simulink model "tvc"  (R2021a)
settings: Solver=VariableStepAuto  StartTime=0.0  StopTime=5  RelTol=1e-3
libraries: simulink_extras x1, simulink x1
settings Model: Creator=shohei  LastModifiedBy=shohei

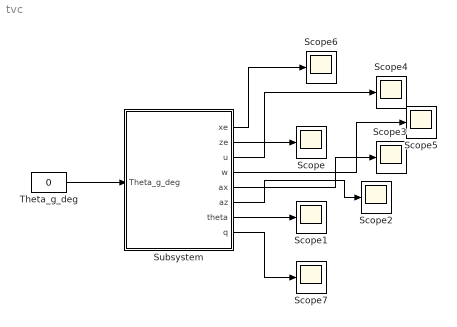
== system tvc ==
  Scope{,1..7} (8 alike) : Scope
  Subsystem : Subsystem
  Theta_g_deg : Constant  Value=0
  wires:
  Theta_g_deg/1 -> Subsystem/1(Theta_g_deg)
  Subsystem/2(ze) -> Scope/1
  Subsystem/7(theta) -> Scope1/1
  Subsystem/6(az) -> Scope2/1
  Subsystem/5(ax) -> Scope3/1
  Subsystem/3(u) -> Scope4/1
  Subsystem/4(w) -> Scope5/1
  Subsystem/1(xe) -> Scope6/1
  Subsystem/8(q) -> Scope7/1

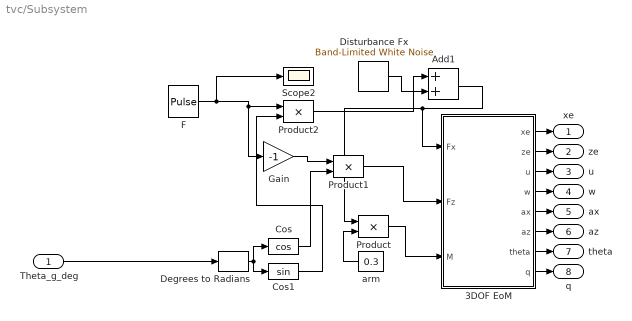
== system tvc/Subsystem ==
  Theta_g_deg : Inport
  3DOF EoM : Subsystem
  Add1 : Sum
  Cos : Trigonometry  Operator=cos
  Cos1 : Trigonometry
  Degrees to Radians : simulink_extras/Transformations/Degrees to Radians
  Disturbance Fx : simulink/Sources/Band-Limited White Noise  Cov=[0.001]  Ts=0.1  seed=[13342]
  F : DiscretePulseGenerator  PulseType=Time based  Amplitude=10  Period=100
  Gain : Gain  Gain=-1
  Product : Product
  Product1 : Product
  Product2 : Product
  Scope2 : Scope
  arm : Constant  Value=0.3
  xe : Outport
  ze : Outport  Port=2
  u : Outport  Port=3
  w : Outport  Port=4
  ax : Outport  Port=5
  az : Outport  Port=6
  theta : Outport  Port=7
  q : Outport  Port=8
  wires:
  3DOF EoM/8(q) -> q/1
  3DOF EoM/6(az) -> az/1
  3DOF EoM/7(theta) -> theta/1
  3DOF EoM/1(xe) -> xe/1
  3DOF EoM/3(u) -> u/1
  3DOF EoM/5(ax) -> ax/1
  Cos1/1 -> Product2/2
  3DOF EoM/4(w) -> w/1
  Product/1 -> 3DOF EoM/3(M)
  3DOF EoM/2(ze) -> ze/1
  Gain/1 -> Product1/1
  Theta_g_deg/1 -> Degrees to Radians/1
  arm/1 -> Product/2
  F/1 -> Gain/1, Product2/1, Scope2/1
  Degrees to Radians/1 -> Cos1/1, Cos/1
  Cos/1 -> Product1/2
  Add1/1 -> Product/1, 3DOF EoM/1(Fx)
  Product2/1 -> Add1/1
  Disturbance Fx/1 -> Add1/2
  Product1/1 -> 3DOF EoM/2(Fz)

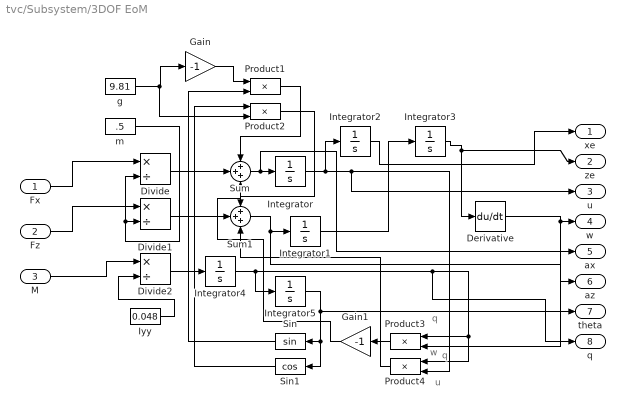
== system tvc/Subsystem/3DOF EoM ==
  note: w
  note: u
  note: q
  note: q
  Fx : Inport
  Fz : Inport  Port=2
  M : Inport  Port=3
  Derivative : Derivative
  Divide : Product  Inputs=*/
  Divide1 : Product  Inputs=*/
  Divide2 : Product  Inputs=*/
  Gain : Gain  Gain=-1
  Gain1 : Gain  Gain=-1
  Integrator{,1..2,4..5} (5 alike) : Integrator
  Integrator3 : Integrator  LimitOutput=on  UpperSaturationLimit=0
  Iyy : Constant  Value=0.048
  Product{1..4} (4 alike) : Product
  Sin : Trigonometry
  Sin1 : Trigonometry  Operator=cos
  Sum : Sum  Inputs=+++
  Sum1 : Sum  Inputs=+++
  g : Constant  Value=9.81
  m : Constant  Value=.5
  xe : Outport
  ze : Outport  Port=2
  u : Outport  Port=3
  w : Outport  Port=4
  ax : Outport  Port=5
  az : Outport  Port=6
  theta : Outport  Port=7
  q : Outport  Port=8
  wires:
  Fz/1 -> Divide1/1
  Gain/1 -> Product1/1
  Divide2/1 -> Integrator4/1
  m/1 -> Divide/2, Divide1/2
  Integrator1/1 -> Integrator3/1
  Product2/1 -> Sum1/1
  Sin/1 -> Product1/2
  Integrator4/1 -> q/1, Product4/1, Product3/1, Integrator5/1
  Fx/1 -> Divide/1
  Product3/1 -> Gain1/1
  M/1 -> Divide2/1
  Product4/1 -> Sum1/3
  Divide1/1 -> Sum1/2
  Sum/1 -> ax/1, Integrator/1
  Product1/1 -> Sum/1
  Integrator5/1 -> theta/1, Sin1/1, Sin/1
  Gain1/1 -> Sum/3
  Iyy/1 -> Divide2/2
  Sin1/1 -> Product2/1
  Divide/1 -> Sum/2
  Integrator/1 -> u/1, Product4/2, Integrator2/1
  Integrator2/1 -> xe/1
  g/1 -> Product2/2, Gain/1
  Sum1/1 -> Integrator1/1, az/1
  Integrator3/1 -> Derivative/1, ze/1
  Derivative/1 -> Product3/2, w/1
